simulink model "test_controller"  (R2018b)
settings: Solver=VariableStepAuto  StartTime=0.0  StopTime=20  FixedStep=Ts  RelTol=1e-3
values from neighbouring files (symbols this model uses):
  A = [0 1 0 0 ... (first row only)    [inverted.m]    (also in kalman_init.m)
  B = [ 0 ... (first row only)    [inverted.m]    (also in kalman_init.m)
  C = [1 0 0 0]    [inverted.m]    (also in kalman_init.m = [1 0 0 0; 0 0 1 0])
  D = zeros(size(C,1),size(B,2))    [inverted.m]    (also in kalman_init.m)
undefined symbols (not defined in the file or in its folder): WLAN
libraries: truetime x4
settings Model: Creator=jiyoj  LastModifiedBy=jiyoj

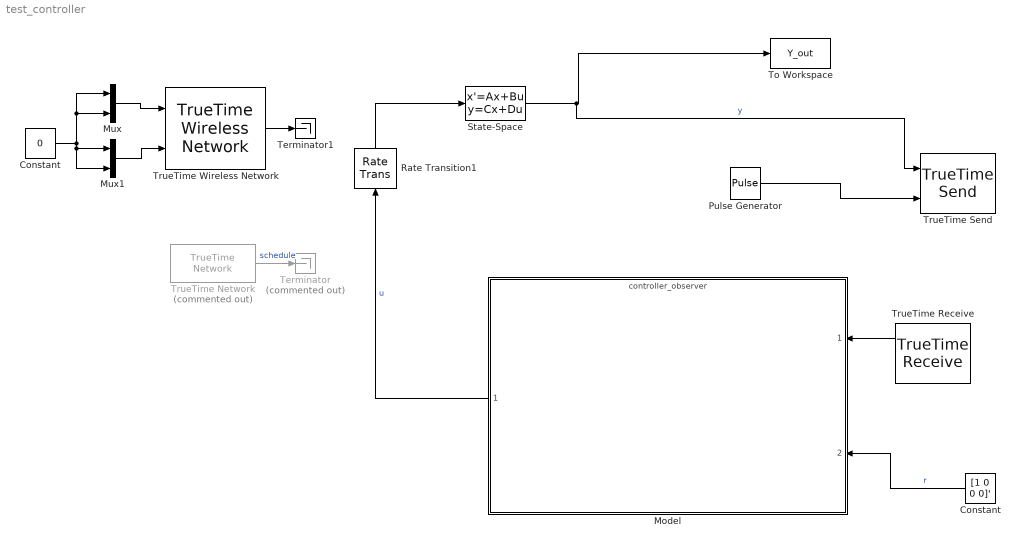
== system test_controller ==
  " Constant" : Constant  Value=[1 0 0 0]'
  Constant : Constant  Value=0
  Model : ModelReference  ModelNameDialog=controller_observer.slx  SimulationMode=Normal  ModelReferenceVersion=1.26
  Mux : Mux  Inputs=2
  Mux1 : Mux  Inputs=2
  Pulse Generator : DiscretePulseGenerator  PulseType=Time based  Period=0.001  PulseWidth=5
  Rate Transition1 : RateTransition
  State-Space : StateSpace  A=A  B=B  C=C  D=D  InitialCondition=0
  Terminator : Terminator  Commented=on
  Terminator1 : Terminator
  To Workspace : ToWorkspace  VariableName=Y_out  SaveFormat=Timeseries  SampleTime=-1
  TrueTime Network : truetime/TrueTime Network  Commented=on  nwtype=CSMA/AMP (CAN)  nwnbr=1  nnodes=1  rate=1000000  minsize=512  lossprob=0  seed=0  bandwidths=[0.5 0.5]  slotsize=512  schedule=[1 1 2]  memsize=80000  buftype=Common buffer  overflow=Retransmit  dynSchedule=0  miniSlotSize=0  NIT=0  QSortMode=FIFO  sync=0  irtSchedule=0  nrtLength=0  nodeGraph=0  scheduleoutput=on
  TrueTime Receive : truetime/TrueTime Receive  nwnbr=1  receiver=1  outdim=2  triggeroutput=on  senderoutput=off  lengthoutput=off  priorityoutput=off  timestampoutput=off  signalpoweroutput=off  msgIDoutput=off
  TrueTime Send : truetime/TrueTime Send  trigger=falling  nwnbr=1  sender=1  indim=2  recsource=internal  receiver=1  lengthsource=internal  length=1000  priosource=internal  prio=1  msgIDsource=internal  msgID=0  dynamicSegment=dynamic
  TrueTime Wireless Network : truetime/TrueTime Wireless  Network  nwtype=802.11b (WLAN)  nwnbr=1  nnodes=2  rate=800000  minsize=272  transpower=20  threshold=-48  use_pathloss_function=default  pathloss=3.5  acktimeout=0.00004  retrylimit=5  error_threshold=0.03  lossprob=0  seed=0  scheduleoutput=on  poweroutput=off
  wires:
  " Constant"/1 -> Model/2  "r"
  Model/1 -> Rate Transition1/1  "u"
  State-Space/1 -> TrueTime Send/1, To Workspace/1  "y"
  Pulse Generator/1 -> TrueTime Send/2
  TrueTime Receive/1 -> Model/1
  Rate Transition1/1 -> State-Space/1
  TrueTime Network/1 -> Terminator/1  "schedule"
  Constant/1 -> Mux1/2, Mux1/1, Mux/2, Mux/1
  Mux1/1 -> TrueTime Wireless Network/2
  Mux/1 -> TrueTime Wireless Network/1
  TrueTime Wireless Network/1 -> Terminator1/1
